simulink model "fpga_block"  (R2020b)
settings: Solver=FixedStepDiscrete  StartTime=0.0  StopTime=5  FixedStep=5e-5  RelTol=1e-3
PostLoadFcn:
  | try
  | cell = struct2cell(dir(fullfile(speedgoatroot_hdlb, 'hdlsrc', 'quadrature', '*.vhd')));
  | addSourceFiles = strjoin(fullfile(cell(2,:),cell(1,:)), ';');
  | hdlset_param('quadrature_example_hdlc/DUT Quadrature', 'IPCoreAdditionalFiles', addSourceFiles);
  | end
libraries: eePwmGenerator x3, simulink x2, pwm_fpgalib x1, quadrature_fpgalib x1, pwm_cpulib x1, quadrature_cpulib x1
settings Model: ModifiedByFormat=Speedgoat GmbH  Creator=Speedgoat GmbH  LastModifiedBy=Speedgoat GmbH
settings DataIOCC: ReturnWorkspaceOutputs=off
settings OptimizationCC: BlockReduction=off  ConditionallyExecuteInputs=off  DefaultParameterBehavior=Inlined
settings DebuggingCC: AlgebraicLoopMsg=error  InheritedTsInSrcMsg=none  SingleTaskRateTransMsg=error  ParameterOverflowMsg=warning  ParameterPrecisionLossMsg=none  PregeneratedLibrarySubsystemCodeDiagnostic=none  ArithmeticOperatorsInVariantConditions=warning
settings HardwareCC: ProdBitPerPointer=32  ProdBitPerSizeT=32  ProdBitPerPtrDiffT=32  ProdLargestAtomicFloat=None  ProdIntDivRoundTo=Undefined  ProdEndianess=Unspecified  ProdWordSize=32  ProdHWDeviceType=ASIC/FPGA->ASIC/FPGA  TargetBitPerPointer=64  TargetBitPerSizeT=64  TargetBitPerPtrDiffT=64  TargetLongLongMode=on  TargetIntDivRoundTo=Zero  TargetEndianess=LittleEndian  TargetWordSize=64  TargetHWDeviceType=Custom Processor->MATLAB Host Computer  ProdEqTarget=off
settings SFSimCC: SimUseLocalCustomCode=off  CustomCodeUndefinedFunction=UseInterfaceOnly
settings RTWCC: RTWUseLocalCustomCode=off

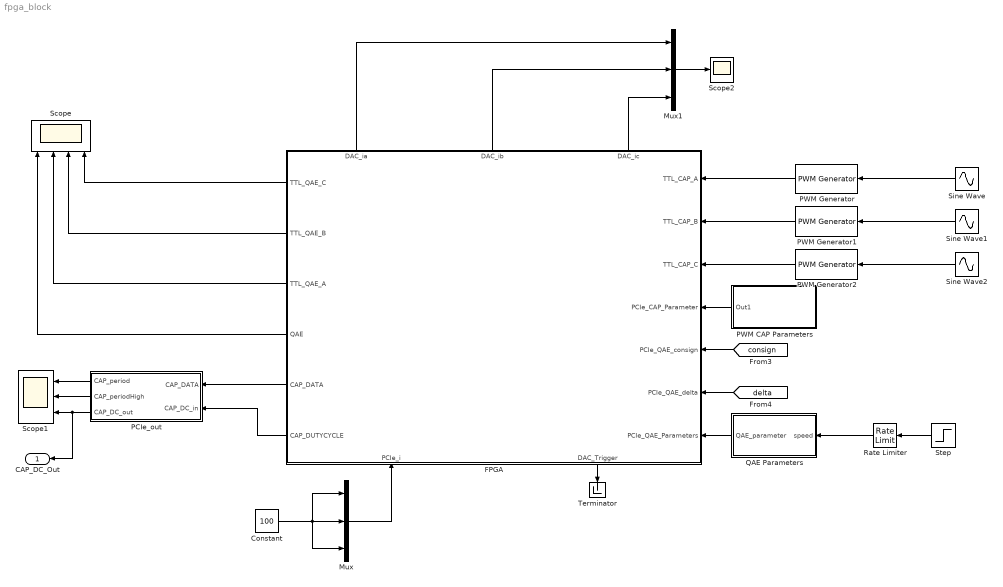
== system fpga_block ==
  Constant : Constant  Value=100  OutDataTypeStr=int16  SampleTime=5e-5
  FPGA : Subsystem
      settings: PortSchema="{\"entries\":[{\"content\":{\"sides\":[{\"content\":{\"connectorIds\":[\"In1\",\"In2\",\"In3\",\"In4\",\"In5\",\"In6\",\"In7\"]},\"type\":\"ConnectorPlacement.EquallySpacedRectSide\",\"uuid\":\"e6984190-0c70-4c87-a85a-93b5ecf8c70e\"},{\"content\":{\"connectorIds\":[\"Out1\",\"Out2\",\"Out3\",\"Out4\",\"Out5\",\"Out6\"],\"side\":\"RIGHT\"},\"type\":\"ConnectorPlacement.EquallySpacedRectSide\",\"uuid\":\"15751016-c591-4c93-a1ea-9b92ed7cff5f\"},{\"content\":{\"connectorIds\":[\"Out8\",\"Out9\",\"Out10\"],\"side\":\"TOP\"},\"type\":\"ConnectorPlacement.EquallySpacedRectSide\",\"uuid\":\"0ed2d626-9fdd-4a40-8e61-e2e65c1699d5\"},{\"content\":{\"connectorIds\":[\"Out7\",\"In8\"],\"side\":\"BOTTOM\"},\"type\":\"ConnectorPlacement.EquallySpacedRectSide\",\"uuid\":\"ca9e0c29-7634-4998-8fab-ad91c1afd2ab\"},{\"content\":{\"connectorIds\":[],\"side\":\"HIDDEN\"},\"type\":\"ConnectorPlacement.EquallySpacedRectSide\",\"uuid\":\"82c879c3-3b90-47c5-9b46-55d1ced3d9d8\"}]},\"type\":\"ConnectorPlacement.EquallySpacedConnector\",\"uuid\":\"f7068230-82ff-4dc7-8776-ae1c0daadd88\"}],\"packageUris\":[\"http://schema.mathworks.com/mf0/Connector/R2020b\"],\"version\":\"1.0\"}"
  Mux : Mux  Inputs=3
  Mux1 : Mux  Inputs=3
  PCIe_out : Subsystem
  PWM CAP Parameters : Subsystem
  PWM Generator : eePwmGenerator/PWM Generator  CarrCount=Up  Tper=0.01  Ts=2e-4
  PWM Generator1 : eePwmGenerator/PWM Generator  CarrCount=Up  Tper=0.01  Ts=2e-4
  PWM Generator2 : eePwmGenerator/PWM Generator  CarrCount=Up  Tper=0.01  Ts=2e-4
  QAE Parameters : Subsystem
  Rate Limiter : RateLimiter  RisingSlewLimit=50  FallingSlewLimit=-50  SampleTimeMode=inherited
  Scope : Scope  NumInputPorts=4
  Scope1 : Scope  NumInputPorts=3
  Scope2 : Scope
  Sine Wave : Sin  Amplitude=0.5  Bias=0.5  Frequency=2*pi
  Sine Wave1 : Sin  Amplitude=0.5  Bias=0.5  Frequency=2*pi  Phase=2*pi/3
  Sine Wave2 : Sin  Amplitude=0.5  Bias=0.5  Frequency=2*pi  Phase=4*pi/3
  Step : Step  Time=0.1  After=100
  Terminator : Terminator
  CAP_DC_Out : Outport  VectorParamsAs1DForOutWhenUnconnected=off
  wires:
  PCIe_out/1(CAP_period) -> Scope1/1
  PCIe_out/2(CAP_periodHigh) -> Scope1/2
  PCIe_out/3(CAP_DC_out) -> Scope1/3, CAP_DC_Out/1
  QAE Parameters/1(QAE_parameter) -> FPGA/7(PCIe_QAE_Parameters)
  [consign] -> FPGA/5(PCIe_QAE_consign)
  [delta] -> FPGA/6(PCIe_QAE_delta)
  PWM Generator/1 -> FPGA/1(TTL_CAP_A)
  PWM Generator1/1 -> FPGA/2(TTL_CAP_B)
  PWM Generator2/1 -> FPGA/3(TTL_CAP_C)
  PWM CAP Parameters/1(Out1) -> FPGA/4(PCIe_CAP_Parameter)
  FPGA/4(QAE) -> Scope/1
  FPGA/3(TTL_QAE_A) -> Scope/2
  FPGA/2(TTL_QAE_B) -> Scope/3
  FPGA/1(TTL_QAE_C) -> Scope/4
  FPGA/5(CAP_DATA) -> PCIe_out/1(CAP_DATA)
  FPGA/6(CAP_DUTYCYCLE) -> PCIe_out/2(CAP_DC_in)
  Rate Limiter/1 -> QAE Parameters/1(speed)
  Step/1 -> Rate Limiter/1
  Sine Wave/1 -> PWM Generator/1
  Sine Wave1/1 -> PWM Generator1/1
  Sine Wave2/1 -> PWM Generator2/1
  Constant/1 -> Mux/3, Mux/2, Mux/1
  Mux1/1 -> Scope2/1
  FPGA/8(DAC_ic) -> Mux1/3
  FPGA/9(DAC_ib) -> Mux1/2
  FPGA/10(DAC_ia) -> Mux1/1
  FPGA/7(DAC_Trigger) -> Terminator/1
  Mux/1 -> FPGA/8(PCIe_i)

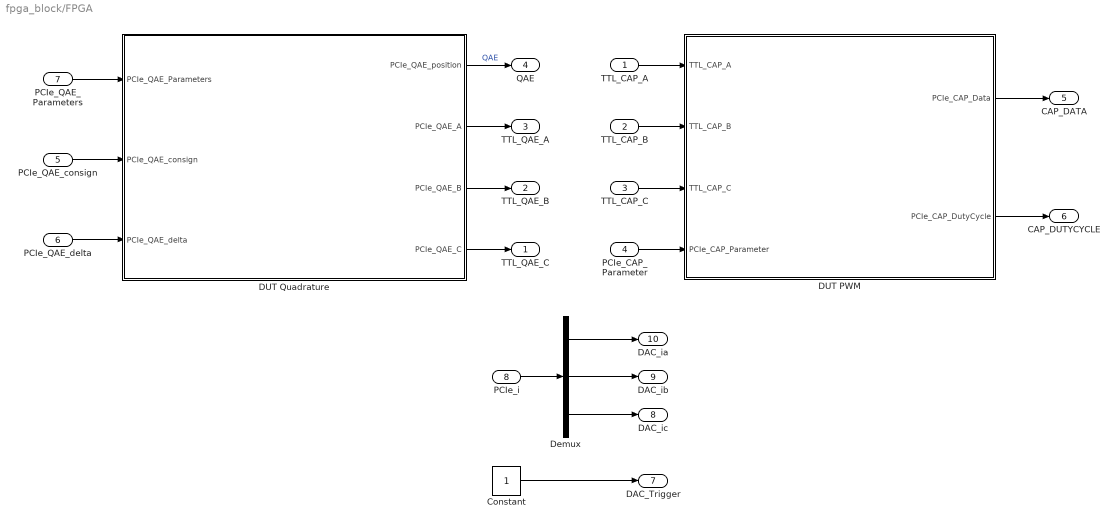
== system fpga_block/FPGA ==
  TTL_CAP_A : Inport
  TTL_CAP_B : Inport  Port=2
  TTL_CAP_C : Inport  Port=3
  PCIe_CAP_Parameter : Inport  Port=4
  PCIe_QAE_consign : Inport  Port=5
  PCIe_QAE_delta : Inport  Port=6
  PCIe_QAE_Parameters : Inport  Port=7
  PCIe_i : Inport  Port=8
  Constant : Constant  OutDataTypeStr=boolean  SampleTime=-1
  DUT PWM : Subsystem
  DUT Quadrature : Subsystem
  Demux : Demux  Outputs=3
  TTL_QAE_C : Outport
  TTL_QAE_B : Outport  Port=2
  TTL_QAE_A : Outport  Port=3
  QAE : Outport  Port=4
  CAP_DATA : Outport  Port=5
  CAP_DUTYCYCLE : Outport  Port=6
  DAC_Trigger : Outport  Port=7
  DAC_ic : Outport  Port=8
  DAC_ib : Outport  Port=9
  DAC_ia : Outport  Port=10
  wires:
  DUT PWM/1(PCIe_CAP_Data) -> CAP_DATA/1
  TTL_CAP_A/1 -> DUT PWM/1(TTL_CAP_A)
  DUT Quadrature/3(PCIe_QAE_B) -> TTL_QAE_B/1
  TTL_CAP_C/1 -> DUT PWM/3(TTL_CAP_C)
  DUT Quadrature/2(PCIe_QAE_A) -> TTL_QAE_A/1
  DUT PWM/2(PCIe_CAP_DutyCycle) -> CAP_DUTYCYCLE/1
  DUT Quadrature/4(PCIe_QAE_C) -> TTL_QAE_C/1
  PCIe_QAE_Parameters/1 -> DUT Quadrature/1(PCIe_QAE_Parameters)
  TTL_CAP_B/1 -> DUT PWM/2(TTL_CAP_B)
  PCIe_QAE_delta/1 -> DUT Quadrature/3(PCIe_QAE_delta)
  PCIe_QAE_consign/1 -> DUT Quadrature/2(PCIe_QAE_consign)
  DUT Quadrature/1(PCIe_QAE_position) -> QAE/1  "QAE"
  PCIe_CAP_Parameter/1 -> DUT PWM/4(PCIe_CAP_Parameter)
  PCIe_i/1 -> Demux/1
  Demux/2 -> DAC_ib/1
  Demux/1 -> DAC_ia/1
  Demux/3 -> DAC_ic/1
  Constant/1 -> DAC_Trigger/1

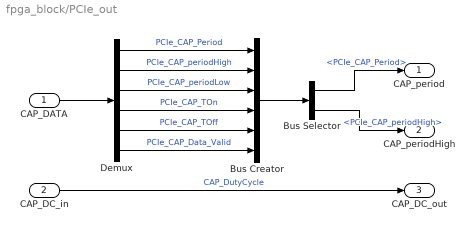
== system fpga_block/PCIe_out ==
  CAP_DATA : Inport
  CAP_DC_in : Inport  Port=2
  Bus Creator : BusCreator  Inputs=6
  Bus Selector : BusSelector  OutputSignals=PCIe_CAP_Period,PCIe_CAP_periodHigh
  Demux : Demux  Outputs=6
  CAP_period : Outport
  CAP_periodHigh : Outport  Port=2
  CAP_DC_out : Outport  Port=3
  wires:
  CAP_DC_in/1 -> CAP_DC_out/1  "CAP_DutyCycle"
  Bus Selector/2 -> CAP_periodHigh/1  "<PCIe_CAP_periodHigh>"
  Bus Selector/1 -> CAP_period/1  "<PCIe_CAP_Period>"
  Demux/6 -> Bus Creator/6  "PCIe_CAP_Data_Valid"
  Demux/3 -> Bus Creator/3  "PCIe_CAP_periodLow"
  Demux/2 -> Bus Creator/2  "PCIe_CAP_periodHigh"
  Demux/4 -> Bus Creator/4  "PCIe_CAP_TOn"
  Bus Creator/1 -> Bus Selector/1
  Demux/1 -> Bus Creator/1  "PCIe_CAP_Period"
  Demux/5 -> Bus Creator/5  "PCIe_CAP_TOff"
  CAP_DATA/1 -> Demux/1

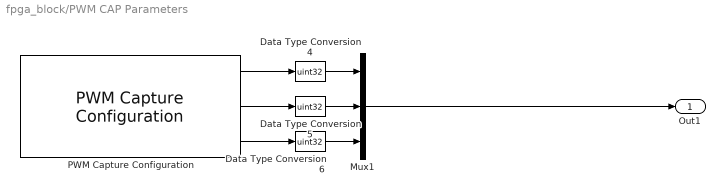
== system fpga_block/PWM CAP Parameters ==
  Data Type Conversion4 : DataTypeConversion  OutDataTypeStr=uint32
  Data Type Conversion5 : DataTypeConversion  OutDataTypeStr=uint32
  Data Type Conversion6 : DataTypeConversion  OutDataTypeStr=uint32
  Mux1 : Mux  Inputs=3
  PWM Capture Configuration : pwm_cpulib/PWM Capture Configuration  FPGA_freq=100e6  n_channels=1  captureMode=High transitions triggered  captureTimeout=0  PWM_pattern_en=off
      settings: SourceProductName=Simulink Real-Time: Speedgoat HDL Blockset
  Out1 : Outport
  wires:
  PWM Capture Configuration/2 -> Data Type Conversion5/1
  Data Type Conversion6/1 -> Mux1/3
  Mux1/1 -> Out1/1
  PWM Capture Configuration/1 -> Data Type Conversion4/1
  Data Type Conversion4/1 -> Mux1/1
  PWM Capture Configuration/3 -> Data Type Conversion6/1
  Data Type Conversion5/1 -> Mux1/2

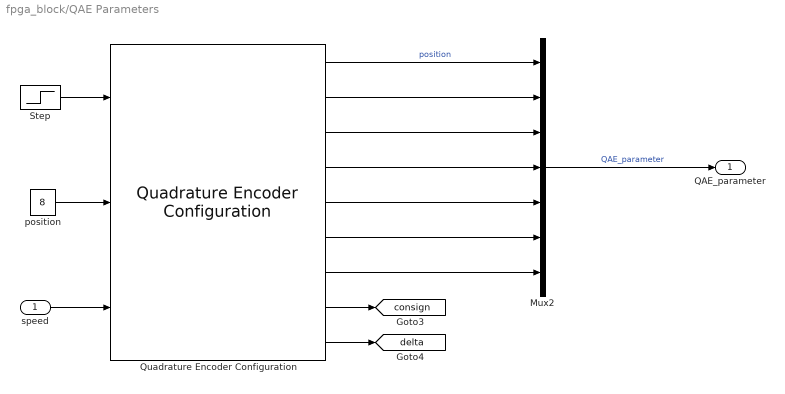
== system fpga_block/QAE Parameters ==
  speed : Inport
  Mux2 : Mux  Inputs=7
  Quadrature Encoder Configuration : quadrature_cpulib/Quadrature Encoder Configuration  fpgaFreq=100e6  n_channels=1  numSeg=[16]  phaseAngle=90  initPos=[0]  freeWheel=on
      settings: SourceProductName=Simulink Real-Time: Speedgoat HDL Blockset
  Step : Step  Time=0.002
  position : Constant  Value=8  SampleTime=-1
  QAE_parameter : Outport
  tag scope: consign=global, delta=global
  wires:
  Quadrature Encoder Configuration/2 -> Mux2/2
  Quadrature Encoder Configuration/5 -> Mux2/5
  Quadrature Encoder Configuration/6 -> Mux2/6
  position/1 -> Quadrature Encoder Configuration/2
  Quadrature Encoder Configuration/8 -> [consign]
  Quadrature Encoder Configuration/3 -> Mux2/3
  Quadrature Encoder Configuration/9 -> [delta]
  speed/1 -> Quadrature Encoder Configuration/3
  Quadrature Encoder Configuration/1 -> Mux2/1  "position"
  Step/1 -> Quadrature Encoder Configuration/1
  Quadrature Encoder Configuration/7 -> Mux2/7
  Quadrature Encoder Configuration/4 -> Mux2/4
  Mux2/1 -> QAE_parameter/1  "QAE_parameter"

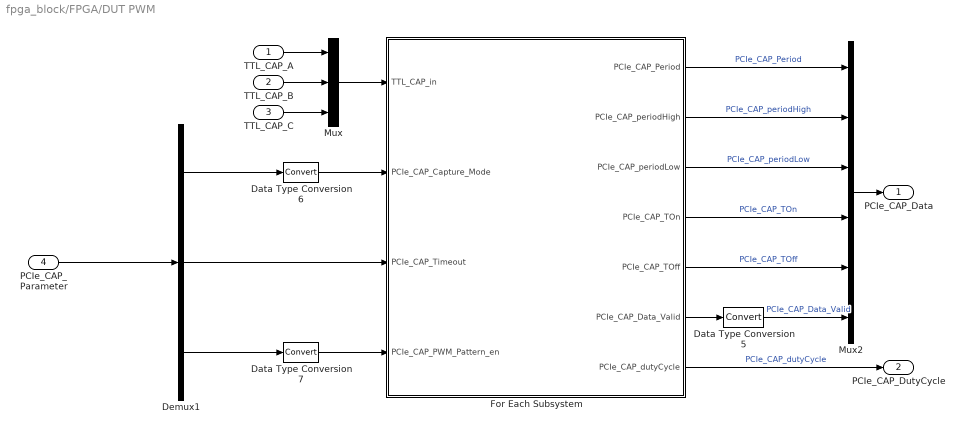
== system fpga_block/FPGA/DUT PWM ==
  TTL_CAP_A : Inport
  TTL_CAP_B : Inport  Port=2
  TTL_CAP_C : Inport  Port=3
  PCIe_CAP_Parameter : Inport  Port=4
  Data Type Conversion5 : DataTypeConversion
  Data Type Conversion6 : DataTypeConversion
  Data Type Conversion7 : DataTypeConversion
  Demux1 : Demux  Outputs=3
  For Each Subsystem : Subsystem  TreatAsAtomicUnit=on
  Mux : Mux  Inputs=3
  Mux2 : Mux  Inputs=6
  PCIe_CAP_Data : Outport  VectorParamsAs1DForOutWhenUnconnected=off
  PCIe_CAP_DutyCycle : Outport  Port=2  VectorParamsAs1DForOutWhenUnconnected=off
  wires:
  Demux1/1 -> Data Type Conversion6/1
  TTL_CAP_A/1 -> Mux/1
  For Each Subsystem/7(PCIe_CAP_dutyCycle) -> PCIe_CAP_DutyCycle/1  "PCIe_CAP_dutyCycle"
  Demux1/2 -> For Each Subsystem/3(PCIe_CAP_Timeout)
  Demux1/3 -> Data Type Conversion7/1
  For Each Subsystem/6(PCIe_CAP_Data_Valid) -> Data Type Conversion5/1
  For Each Subsystem/5(PCIe_CAP_TOff) -> Mux2/5  "PCIe_CAP_TOff"
  For Each Subsystem/4(PCIe_CAP_TOn) -> Mux2/4  "PCIe_CAP_TOn"
  For Each Subsystem/3(PCIe_CAP_periodLow) -> Mux2/3  "PCIe_CAP_periodLow"
  For Each Subsystem/1(PCIe_CAP_Period) -> Mux2/1  "PCIe_CAP_Period"
  For Each Subsystem/2(PCIe_CAP_periodHigh) -> Mux2/2  "PCIe_CAP_periodHigh"
  Mux/1 -> For Each Subsystem/1(TTL_CAP_in)
  TTL_CAP_B/1 -> Mux/2
  Mux2/1 -> PCIe_CAP_Data/1
  Data Type Conversion5/1 -> Mux2/6  "PCIe_CAP_Data_Valid"
  PCIe_CAP_Parameter/1 -> Demux1/1
  Data Type Conversion6/1 -> For Each Subsystem/2(PCIe_CAP_Capture_Mode)
  Data Type Conversion7/1 -> For Each Subsystem/4(PCIe_CAP_PWM_Pattern_en)
  TTL_CAP_C/1 -> Mux/3

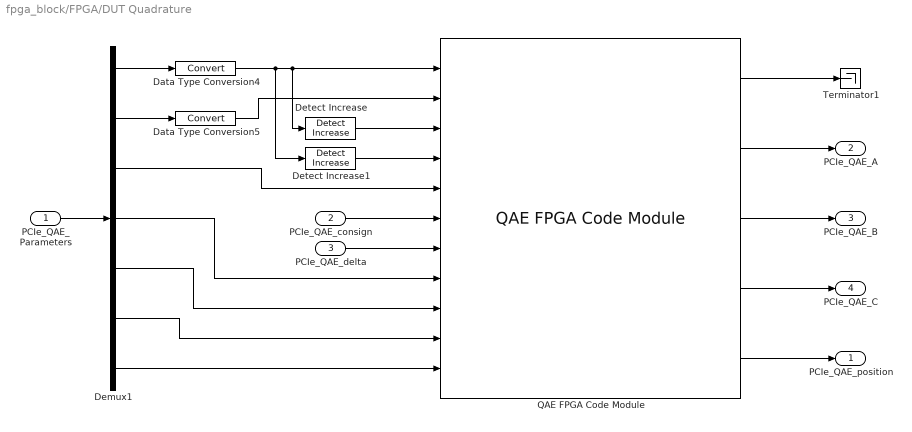
== system fpga_block/FPGA/DUT Quadrature ==
  PCIe_QAE_Parameters : Inport
  PCIe_QAE_consign : Inport  Port=2  OutDataTypeStr=uint32  PortDimensions=1
  PCIe_QAE_delta : Inport  Port=3  PortDimensions=1
  Data Type Conversion4 : DataTypeConversion
  Data Type Conversion5 : DataTypeConversion
  Demux1 : Demux  Outputs=7
  Detect Increase : simulink/Logic and Bit Operations/Detect Increase  vinit=0.0  OutDataTypeStr=boolean
  Detect Increase1 : simulink/Logic and Bit Operations/Detect Increase  vinit=0.0  OutDataTypeStr=boolean
  QAE FPGA Code Module : quadrature_fpgalib/QAE FPGA Code Module  SystemSampleTime=-1  VariantActivationTime=update diagram  Latency=0  AutoFrameSizeCalculation=off
      settings: SourceProductName=Simulink Real-Time: Speedgoat Functionality Package
  Terminator1 : Terminator
  PCIe_QAE_position : Outport  VectorParamsAs1DForOutWhenUnconnected=off
  PCIe_QAE_A : Outport  Port=2  VectorParamsAs1DForOutWhenUnconnected=off
  PCIe_QAE_B : Outport  Port=3  VectorParamsAs1DForOutWhenUnconnected=off
  PCIe_QAE_C : Outport  Port=4  VectorParamsAs1DForOutWhenUnconnected=off
  wires:
  QAE FPGA Code Module/5 -> PCIe_QAE_position/1
  Detect Increase1/1 -> QAE FPGA Code Module/4
  Detect Increase/1 -> QAE FPGA Code Module/3
  QAE FPGA Code Module/4 -> PCIe_QAE_C/1
  QAE FPGA Code Module/2 -> PCIe_QAE_A/1
  QAE FPGA Code Module/3 -> PCIe_QAE_B/1
  PCIe_QAE_delta/1 -> QAE FPGA Code Module/7
  QAE FPGA Code Module/1 -> Terminator1/1
  PCIe_QAE_consign/1 -> QAE FPGA Code Module/6
  Demux1/1 -> Data Type Conversion4/1
  Demux1/2 -> Data Type Conversion5/1
  Demux1/3 -> QAE FPGA Code Module/5
  Demux1/4 -> QAE FPGA Code Module/8
  Demux1/5 -> QAE FPGA Code Module/9
  PCIe_QAE_Parameters/1 -> Demux1/1
  Data Type Conversion4/1 -> Detect Increase1/1, QAE FPGA Code Module/1, Detect Increase/1
  Data Type Conversion5/1 -> QAE FPGA Code Module/2
  Demux1/6 -> QAE FPGA Code Module/10
  Demux1/7 -> QAE FPGA Code Module/11

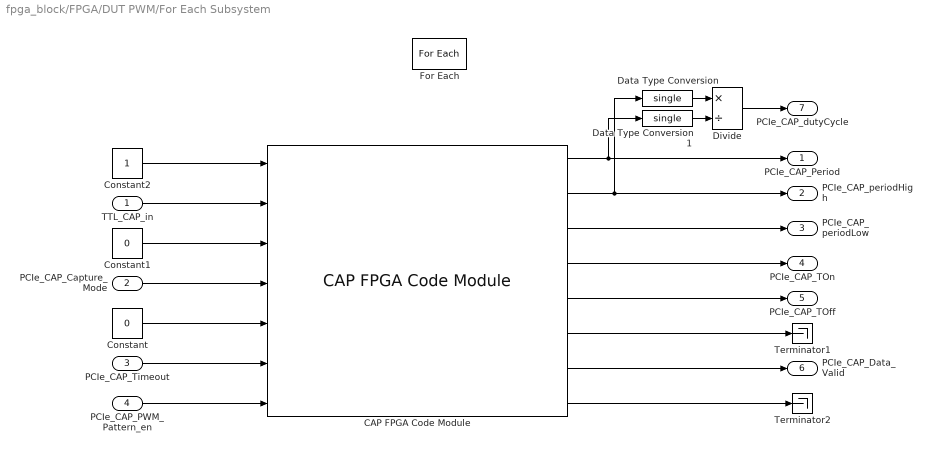
== system fpga_block/FPGA/DUT PWM/For Each Subsystem ==
  TTL_CAP_in : Inport  Partition=on  PartitionDimension=1  PartitionWidth=1  PartitionOffset=0
  PCIe_CAP_Capture_Mode : Inport  Port=2
  PCIe_CAP_Timeout : Inport  Port=3
  PCIe_CAP_PWM_Pattern_en : Inport  Port=4
  CAP FPGA Code Module : pwm_fpgalib/CAP FPGA Code Module  SystemSampleTime=-1  VariantActivationTime=update diagram  Latency=0  AutoFrameSizeCalculation=off
      settings: SourceProductName=Simulink Real-Time: Speedgoat Functionality Package
  Constant : Constant  Value=0  OutDataTypeStr=Inherit: Inherit via back propagation  SampleTime=-1
  Constant1 : Constant  Value=0  OutDataTypeStr=Inherit: Inherit via back propagation  SampleTime=-1
  Constant2 : Constant  OutDataTypeStr=Inherit: Inherit via back propagation  SampleTime=-1
  Data Type Conversion : DataTypeConversion  OutMin=0  OutDataTypeStr=single
  Data Type Conversion1 : DataTypeConversion  OutMin=0  OutDataTypeStr=single  LockScale=on
  Divide : Product  Inputs=*/  RndMeth=Zero  SaturateOnIntegerOverflow=on
  For Each : ForEach  DisableCoverage=on
  Terminator1 : Terminator
  Terminator2 : Terminator
  PCIe_CAP_Period : Outport  ConcatenationDimension=2  VectorParamsAs1DForOutWhenUnconnected=off
  PCIe_CAP_periodHigh : Outport  Port=2  ConcatenationDimension=2  VectorParamsAs1DForOutWhenUnconnected=off
  PCIe_CAP_periodLow : Outport  Port=3  ConcatenationDimension=2  VectorParamsAs1DForOutWhenUnconnected=off
  PCIe_CAP_TOn : Outport  Port=4  ConcatenationDimension=2  VectorParamsAs1DForOutWhenUnconnected=off
  PCIe_CAP_TOff : Outport  Port=5  ConcatenationDimension=2  VectorParamsAs1DForOutWhenUnconnected=off
  PCIe_CAP_Data_Valid : Outport  Port=6  ConcatenationDimension=2  VectorParamsAs1DForOutWhenUnconnected=off
  PCIe_CAP_dutyCycle : Outport  Port=7  ConcatenationDimension=2  VectorParamsAs1DForOutWhenUnconnected=off
  wires:
  Data Type Conversion/1 -> Divide/1
  Divide/1 -> PCIe_CAP_dutyCycle/1
  Constant1/1 -> CAP FPGA Code Module/3
  PCIe_CAP_Capture_Mode/1 -> CAP FPGA Code Module/4
  Constant/1 -> CAP FPGA Code Module/5
  TTL_CAP_in/1 -> CAP FPGA Code Module/2
  PCIe_CAP_Timeout/1 -> CAP FPGA Code Module/6
  PCIe_CAP_PWM_Pattern_en/1 -> CAP FPGA Code Module/7
  Constant2/1 -> CAP FPGA Code Module/1
  CAP FPGA Code Module/3 -> PCIe_CAP_periodLow/1
  CAP FPGA Code Module/8 -> Terminator2/1
  CAP FPGA Code Module/5 -> PCIe_CAP_TOff/1
  CAP FPGA Code Module/6 -> Terminator1/1
  CAP FPGA Code Module/2 -> PCIe_CAP_periodHigh/1, Data Type Conversion/1
  CAP FPGA Code Module/7 -> PCIe_CAP_Data_Valid/1
  CAP FPGA Code Module/1 -> PCIe_CAP_Period/1, Data Type Conversion1/1
  CAP FPGA Code Module/4 -> PCIe_CAP_TOn/1
  Data Type Conversion1/1 -> Divide/2
